simulink model "SLIP_angle"  (R2015a)
settings: Solver=ode45  StartTime=0.0  StopTime=10.0  RelTol=1e-3
settings Model: Creator=BML  LastModifiedBy=BML

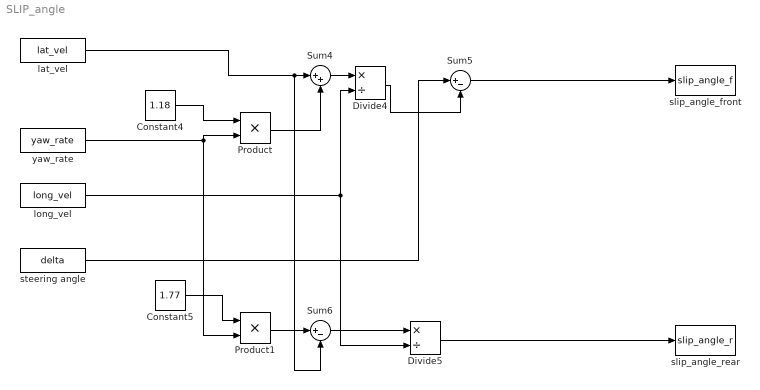
== system SLIP_angle ==
  Constant4 : Constant  Value=1.18
  Constant5 : Constant  Value=1.77
  Divide4 : Product  Inputs=*/
  Divide5 : Product  Inputs=*/
  Product : Product
  Product1 : Product
  Sum4 : Sum  Inputs=|++
  Sum5 : Sum  Inputs=|+-
  Sum6 : Sum  Inputs=|+-
  lat_vel : FromWorkspace  VariableName=lat_vel  SampleTime=0
  long_vel : FromWorkspace  VariableName=long_vel  SampleTime=0
  slip_angle_front : ToWorkspace  VariableName=slip_angle_f  SaveFormat=Timeseries  SampleTime=-1
  slip_angle_rear : ToWorkspace  VariableName=slip_angle_r  SaveFormat=Timeseries  SampleTime=-1
  steering angle : FromWorkspace  VariableName=delta  SampleTime=0
  yaw_rate : FromWorkspace  VariableName=yaw_rate  SampleTime=0
  wires:
  Constant4/1 -> Product/1
  yaw_rate/1 -> Product1/2, Product/2
  Product/1 -> Sum4/2
  Sum4/1 -> Divide4/1
  long_vel/1 -> Divide5/2, Divide4/2
  Sum5/1 -> slip_angle_front/1
  steering angle/1 -> Sum5/1
  Divide4/1 -> Sum5/2
  Constant5/1 -> Product1/1
  Product1/1 -> Sum6/1
  lat_vel/1 -> Sum6/2, Sum4/1
  Sum6/1 -> Divide5/1
  Divide5/1 -> slip_angle_rear/1
